simulink model "compliance_adjusting_controller"  (R2020b)
settings: Solver=VariableStepAuto  StartTime=0.0  StopTime=60  RelTol=1e-3
values from neighbouring files (symbols this model uses):
  alpha = 0.001    [compliance_PLUS_energy_setup.m]    (also in compliance_adjusting_setup.m = 200; hyperbole_test.m = 1000)
  b0 = 2 * sqrt(k0 * m_R)    [compliance_PLUS_energy_setup.m]    (also in compliance_adjusting_setup.m = 20; energy_aware_setup.m = 20; optim_criteria.m = 0.2; plot_meshes.m = 0.2)
  C_max = 10    [compliance_PLUS_energy_setup.m]    (also in compliance_adjusting_setup.m = 1)
  F_cmax = 5    [compliance_PLUS_energy_setup.m]    (also in compliance_adjusting_setup.m)
  k0 = 20    [compliance_PLUS_energy_setup.m]    (also in compliance_adjusting_setup.m = 100; energy_aware_setup.m = 100; optim_criteria.m = 1; plot_meshes.m = 1)
  km = 100    [compliance_PLUS_energy_setup.m]    (also in compliance_adjusting_setup.m; energy_aware_setup.m; setup.m)
  m_R = 1    [compliance_PLUS_energy_setup.m]    (also in compliance_adjusting_setup.m; energy_aware_setup.m; setup.m)
  sigma = 0    [compliance_PLUS_energy_setup.m]    (also in compliance_adjusting_setup.m)
  T = 1/30    (= 0.0333333333333)    [compliance_PLUS_energy_setup.m]    (also in compliance_adjusting_setup.m)
  t_collision = 20    [compliance_PLUS_energy_setup.m]    (also in compliance_adjusting_setup.m; energy_aware_setup.m; setup.m)
  t_init = 2    [compliance_PLUS_energy_setup.m]    (also in compliance_adjusting_setup.m; energy_aware_setup.m; setup.m)
  x_O = 0.5    [compliance_PLUS_energy_setup.m]    (also in compliance_adjusting_setup.m; energy_aware_setup.m; setup.m)
  x_R = 0    [compliance_PLUS_energy_setup.m]    (also in compliance_adjusting_setup.m; energy_aware_setup.m; setup.m)
libraries: neural x1
settings Model: Creator=kika  LastModifiedBy=kika

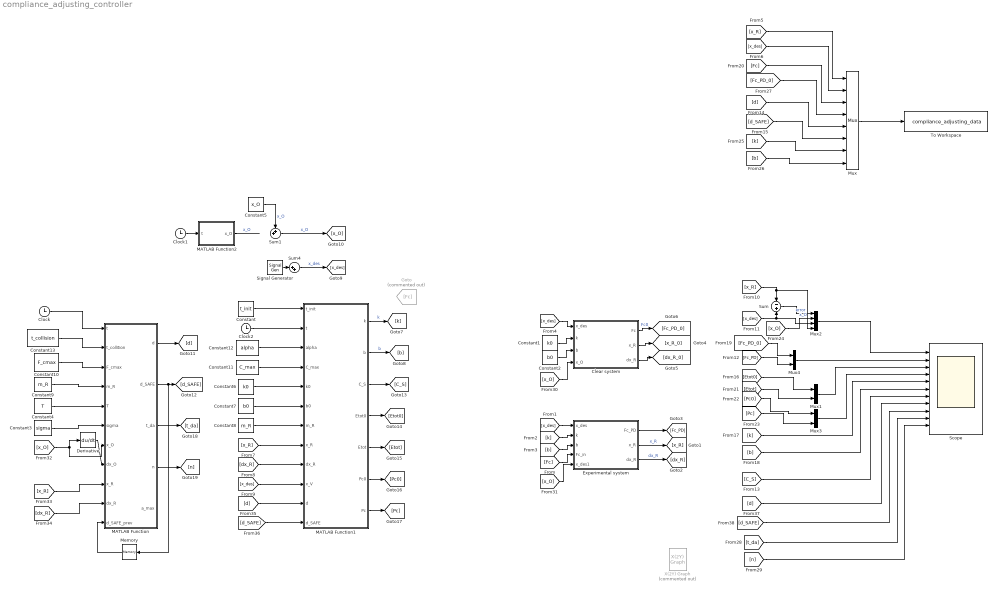
== system compliance_adjusting_controller ==
  Clear system : Subsystem
  Clock : Clock
  Clock1 : Clock
  Clock2 : Clock
  Constant : Constant  Value=t_init
  Constant1 : Constant  Value=k0
  Constant10 : Constant  Value=F_cmax
  Constant11 : Constant  Value=C_max
  Constant12 : Constant  Value=alpha
  Constant13 : Constant  Value=t_collision
  Constant2 : Constant  Value=b0
  Constant3 : Constant  Value=sigma
  Constant4 : Constant  Value=T
  Constant5 : Constant  Value=x_O
  Constant6 : Constant  Value=k0
  Constant7 : Constant  Value=b0
  Constant8 : Constant  Value=m_R
  Constant9 : Constant  Value=m_R
  Derivative : Derivative
  Experimental system : Subsystem
  Goto : Goto  Commented=on  GotoTag=Fc
  MATLAB Function : MATLAB Function  TreatAsAtomicUnit=on
  MATLAB Function1 : MATLAB Function  TreatAsAtomicUnit=on
  MATLAB Function2 : MATLAB Function  TreatAsAtomicUnit=on
  Memory : Memory
  Mux : Mux  Inputs=8
  Mux1 : Mux  Inputs=2
  Mux2 : Mux
  Mux3 : Mux  Inputs=2
  Mux4 : Mux  Inputs=2
  Scope : Scope  NumInputPorts=11
  Signal Generator : SignalGenerator  Frequency=0.5  Units=rad/sec
  Sum : Sum  Inputs=-+
  Sum1 : Sum  Inputs=++|
  Sum4 : Sum  Inputs=|++
  To Workspace : ToWorkspace  VariableName=compliance_adjusting_data  SaveFormat=Timeseries  SampleTime=-1
  X(2Y) Graph : neural/Control Systems/X(2Y)  Graph  Commented=on  xmin=0  xmax=5  ymin=21  ymax=22  st=-1
      settings: SourceProductBaseCode=NN
  wires:
  Constant7/1 -> MATLAB Function1/6(b0)
  MATLAB Function1/1(k) -> [k]  "k"
  Constant8/1 -> MATLAB Function1/7(m_R)
  Constant6/1 -> MATLAB Function1/5(k0)
  Clock2/1 -> MATLAB Function1/2(t)
  MATLAB Function1/2(b) -> [b]  "b"
  Signal Generator/1 -> Sum4/1
  Constant/1 -> MATLAB Function1/1(t_init)
  [Fc] -> Experimental system/4(Fc_in)
  [x_des] -> Experimental system/1(x_des)
  Experimental system/2(x_R) -> [x_R]  "x_R"
  Experimental system/3(dx_R) -> [dx_R]  "dx_R"
  Experimental system/1(Fc_PD) -> [Fc_PD]
  Clear system/1(Fc) -> [Fc_PD_0]  "Fc0"
  Clear system/2(x_R) -> [x_R_0]
  Clear system/3(dx_R) -> [dx_R_0]
  [k] -> Experimental system/2(k)
  [b] -> Experimental system/3(b)
  [x_des] -> Clear system/1(x_des)
  Constant1/1 -> Clear system/2(k)
  Constant2/1 -> Clear system/3(b)
  [dx_R] -> MATLAB Function1/9(dx_R)
  [x_R] -> MATLAB Function1/8(x_R)
  Sum4/1 -> [x_des]  "x_des"
  [x_des] -> MATLAB Function1/10(x_V)
  [x_R] -> Mux2/4, Sum/1
  [x_des] -> Mux2/3, Sum/2
  Mux2/1 -> Scope/1
  [Fc_PD] -> Mux4/2
  [k] -> Scope/5
  [b] -> Scope/6
  [Fc_PD_0] -> Mux4/1
  Mux4/1 -> Scope/2
  Sum/1 -> Mux2/1  "error"
  Mux/1 -> To Workspace/1
  [x_O] -> Experimental system/5(x_des1)
  [x_O] -> Clear system/4(x_O)
  [x_O] -> Derivative/1, MATLAB Function/7(x_O)
  [x_R] -> MATLAB Function/9(x_R)
  [dx_R] -> MATLAB Function/10(dx_R)
  Derivative/1 -> MATLAB Function/8(dx_O)
  Constant3/1 -> MATLAB Function/6(sigma)
  Constant4/1 -> MATLAB Function/5(T)
  Constant9/1 -> MATLAB Function/4(m_R)
  Constant10/1 -> MATLAB Function/3(F_cmax)
  Constant11/1 -> MATLAB Function1/4(C_max)
  Constant12/1 -> MATLAB Function1/3(alpha)
  [d_SAFE] -> MATLAB Function1/12(d_SAFE)
  [d] -> MATLAB Function1/11(d)
  MATLAB Function/1(d) -> [d]
  MATLAB Function/2(d_SAFE) -> Memory/1, [d_SAFE]
  Constant13/1 -> MATLAB Function/2(t_collition)
  Clock/1 -> MATLAB Function/1(t)
  MATLAB Function1/3(C_S) -> [C_S]
  [C_S] -> Scope/7
  [d_SAFE] -> Mux/6
  [Fc_PD_0] -> Mux/4
  [d] -> Mux/5
  [k] -> Mux/7
  [b] -> Mux/8
  [Fc] -> Mux/3
  [x_des] -> Mux/2
  [x_R] -> Mux/1
  [d] -> Scope/8
  [d_SAFE] -> Scope/9
  Mux1/1 -> Scope/3
  Mux3/1 -> Scope/4
  MATLAB Function1/7(Pc) -> [Pc]
  MATLAB Function1/6(Pc0) -> [Pc0]
  MATLAB Function1/5(Etot) -> [Etot]
  MATLAB Function1/4(Etot0) -> [Etot0]
  [Etot0] -> Mux1/1
  [Etot] -> Mux1/2
  [Pc0] -> Mux3/1
  [Pc] -> Mux3/2
  Constant5/1 -> Sum1/1  "x_O"
  [x_O] -> Mux2/2  "x_O"
  Sum1/1 -> [x_O]  "x_O"
  MATLAB Function2/1(x_O) -> ?  "x_O"
  Clock1/1 -> MATLAB Function2/1(t)
  Memory/1 -> MATLAB Function/11(d_SAFE_prev)
  MATLAB Function/3(t_da) -> [t_da]
  MATLAB Function/4(n) -> [n]
  [t_da] -> Scope/10
  [n] -> Scope/11

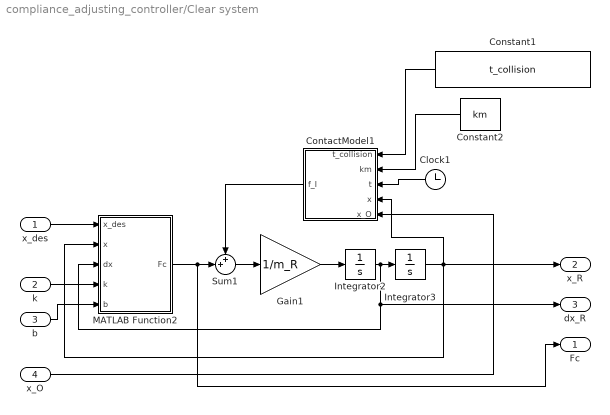
== system compliance_adjusting_controller/Clear system ==
  x_des : Inport
  k : Inport  Port=2
  b : Inport  Port=3
  x_O : Inport  Port=4
  Clock1 : Clock
  Constant1 : Constant  Value=t_collision
  Constant2 : Constant  Value=km
  ContactModel1 : MATLAB Function  TreatAsAtomicUnit=on
  Gain1 : Gain  Gain=1/m_R
  Integrator2 : Integrator
  Integrator3 : Integrator  InitialCondition=x_R
  MATLAB Function2 : MATLAB Function  TreatAsAtomicUnit=on
  Sum1 : Sum  Inputs=++|
  Fc : Outport
  x_R : Outport  Port=2
  dx_R : Outport  Port=3
  wires:
  k/1 -> MATLAB Function2/4(k)
  ContactModel1/1(f_I) -> Sum1/1
  Clock1/1 -> ContactModel1/3(t)
  Integrator3/1 -> x_R/1, ContactModel1/4(x), MATLAB Function2/2(x)
  x_des/1 -> MATLAB Function2/1(x_des)
  b/1 -> MATLAB Function2/5(b)
  Sum1/1 -> Gain1/1
  x_O/1 -> ContactModel1/5(x_O)
  Gain1/1 -> Integrator2/1
  MATLAB Function2/1(Fc) -> Fc/1, Sum1/2
  Integrator2/1 -> dx_R/1, MATLAB Function2/3(dx), Integrator3/1
  Constant1/1 -> ContactModel1/1(t_collision)
  Constant2/1 -> ContactModel1/2(km)

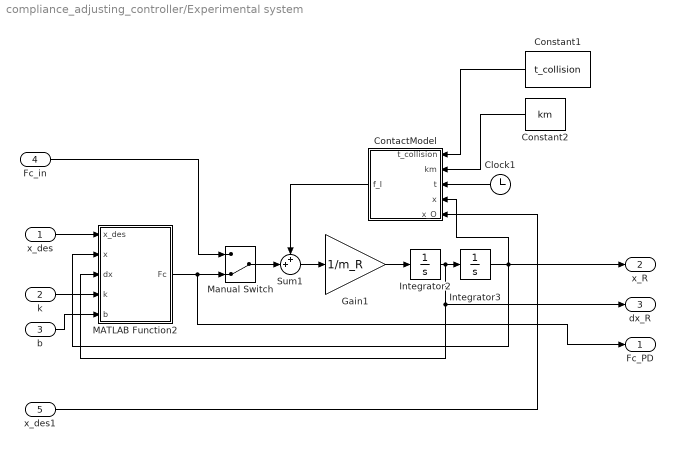
== system compliance_adjusting_controller/Experimental system ==
  x_des : Inport
  k : Inport  Port=2
  b : Inport  Port=3
  Fc_in : Inport  Port=4
  x_des1 : Inport  Port=5
  Clock1 : Clock
  Constant1 : Constant  Value=t_collision
  Constant2 : Constant  Value=km
  ContactModel : MATLAB Function  TreatAsAtomicUnit=on
  Gain1 : Gain  Gain=1/m_R
  Integrator2 : Integrator
  Integrator3 : Integrator  InitialCondition=x_R
  MATLAB Function2 : MATLAB Function  TreatAsAtomicUnit=on
  Manual Switch : ManualSwitch  CurrentSetting=0
  Sum1 : Sum  Inputs=++|
  Fc_PD : Outport
  x_R : Outport  Port=2
  dx_R : Outport  Port=3
  wires:
  k/1 -> MATLAB Function2/4(k)
  ContactModel/1(f_I) -> Sum1/1
  Clock1/1 -> ContactModel/3(t)
  Integrator3/1 -> x_R/1, ContactModel/4(x), MATLAB Function2/2(x)
  x_des/1 -> MATLAB Function2/1(x_des)
  b/1 -> MATLAB Function2/5(b)
  Sum1/1 -> Gain1/1
  x_des1/1 -> ContactModel/5(x_O)
  Gain1/1 -> Integrator2/1
  MATLAB Function2/1(Fc) -> Manual Switch/2, Fc_PD/1
  Integrator2/1 -> dx_R/1, MATLAB Function2/3(dx), Integrator3/1
  Constant1/1 -> ContactModel/1(t_collision)
  Constant2/1 -> ContactModel/2(km)
  Fc_in/1 -> Manual Switch/1
  Manual Switch/1 -> Sum1/2

== matlab function compliance_adjusting_controller/MATLAB Function ==
  data: t input; t_collition input; F_cmax input; m_R input; T input; sigma input; x_O input; dx_O input; d output; x_R input; dx_R input; d_SAFE output; t_da output; n output; a_max output; d_SAFE_prev input
function [d, d_SAFE, t_da, n, a_max] = SENSING(t, t_collition, F_cmax, m_R, T, sigma, x_O, dx_O, x_R, dx_R, d_SAFE_prev)

    
    d = 0.1;
    d_SAFE = 0;
    
    
    a_max = F_cmax / m_R;
    t_da = abs((dx_R - dx_O) / a_max);
%     n = ceil(t_da*10)/10 / T;
    n = ceil(t_da / T);
    
    
   
    if t > t_collition
        if x_R <= x_O
            d = abs(x_R - x_O);
        else
            d = 0;
        end
        
        % d_SAFE calculation (deaceleration path length using F_cmax)
        d_SAFE = abs(dx_R - dx_O) * n * T;
%         d_SAFE = 0.4 * d_SAFE + 0.6 * d_SAFE_prev;
%         d_SAFE = 0.1;
    %     d_SAFE = abs(dx_R - dx_O) * n * T + 3 * sigma;
    end

== matlab function compliance_adjusting_controller/MATLAB Function2 ==
  data: t input; x_O output
function x_O = fcn(t)

x_O = sin(0.5 * t + pi);

== matlab function compliance_adjusting_controller/Experimental system/ContactModel ==
  data: t_collision input; km input; t input; f_I output; x input; x_O input
function f_I = fcn(t_collision, km, t, x, x_O)


f_I = 0;

if t > t_collision
    if x > x_O
        f_I = km * (x_O - x);
    end
end

== matlab function compliance_adjusting_controller/Experimental system/MATLAB Function2 ==
  data: x_des input; Fc output; x input; dx input; k input; b input
function Fc = fcn(x_des, x, dx, k, b)

Fc = k * (x_des - x) - b * dx;

== matlab function compliance_adjusting_controller/MATLAB Function1 ==
  data: t_init input; t input; alpha input; C_max input; k0 input; b0 input; m_R input; x_R input; k output; b output; dx_R input; x_V input; d input; d_SAFE input; C_S output; Etot0 output; Etot output; Pc0 output; Pc output
function [k, b, C_S, Etot0, Etot, Pc0, Pc] = compliance(t_init, t, alpha, C_max, k0, b0, m_R, x_R, dx_R, x_V, d, d_SAFE)
    
    k = k0;
    b = b0;
    
    e = x_V - x_R;
    
    Etot0 = 0.5 * m_R * dx_R^2 + 0.5 * k * e^2;
    Pc0 = (k * e - b * dx_R) * dx_R;
    
    C_0 = 1 / k0;

    beta = 1 / C_max;
    C_S = 0;
    if d <= d_SAFE
        C_S = 1 / (alpha * d + beta);
    
        k = 1 / (C_0 + C_S);

        % critical damping
        b = 2 * sqrt(k * m_R);
    end
    
    Etot = 0.5 * m_R * dx_R^2 + 0.5 * k * e^2;
    Pc = (k * e - b * dx_R) * dx_R;

== matlab function compliance_adjusting_controller/Clear system/MATLAB Function2 ==
  data: x_des input; Fc output; x input; dx input; k input; b input
function Fc = fcn(x_des, x, dx, k, b)

Fc = k * (x_des - x) - b * dx;

== matlab function compliance_adjusting_controller/Clear system/ContactModel1 ==
  data: t_collision input; km input; t input; f_I output; x input; x_O input
function f_I = fcn(t_collision, km, t, x, x_O)


f_I = 0;

if t > t_collision
    if x > x_O
        f_I = km * (x_O - x);
    end
end
